simulink model "Assignment1"  (R2017b)
settings: Solver=FixedStepAuto  StartTime=0.0  StopTime=6  FixedStep=1e-3  RelTol=1e-3  EnableMultiTasking=on
undefined symbols (not defined in the file): D10, D11, D12, D2, D3, D4, D7, D8, D9, PTA0, PTA1, PTB23, PTB9, PTC3, PTC4, PTD0, PTD2, PTD3
libraries: frdmk64flib x12
settings Model: ExtModeTrigDuration=5  Creator=iannanla  LastModifiedBy=iannanla
settings DataIOCC: InspectSignalLogs=on
settings OptimizationCC: PassReuseOutputArgsAs=Individual arguments  MaxStackSize=64
settings DebuggingCC: ParameterTunabilityLossMsg=error
settings HardwareCC: ProdBitPerPointer=32  ProdBitPerSizeT=32  ProdBitPerPtrDiffT=32  ProdLargestAtomicInteger=Long  ProdLargestAtomicFloat=Double  ProdWordSize=32  ProdHWDeviceType=ARM Compatible->ARM Cortex
settings SFSimCC: MATLABDynamicMemAlloc=off
settings RTWCC: SystemTargetFile=ert.tlc  HardwareBoard=NXP FRDM-K64F  TemplateMakefile=ert_default_tmf  GenerateReport=on  Toolchain=GNU Tools for ARM Embedded Processors  IncludeHyperlinkInReport=on  LaunchReport=on  GenerateTraceInfo=on  GenerateTraceReport=on  GenerateTraceReportSl=on  GenerateTraceReportSf=on  GenerateTraceReportEml=on
settings CodeAppCC: ForceParamTrailComments=on  IgnoreCustomStorageClasses=off  OperatorAnnotations=on  SimulinkDataObjDesc=on  SFDataObjDesc=on  InsertBlockDesc=on

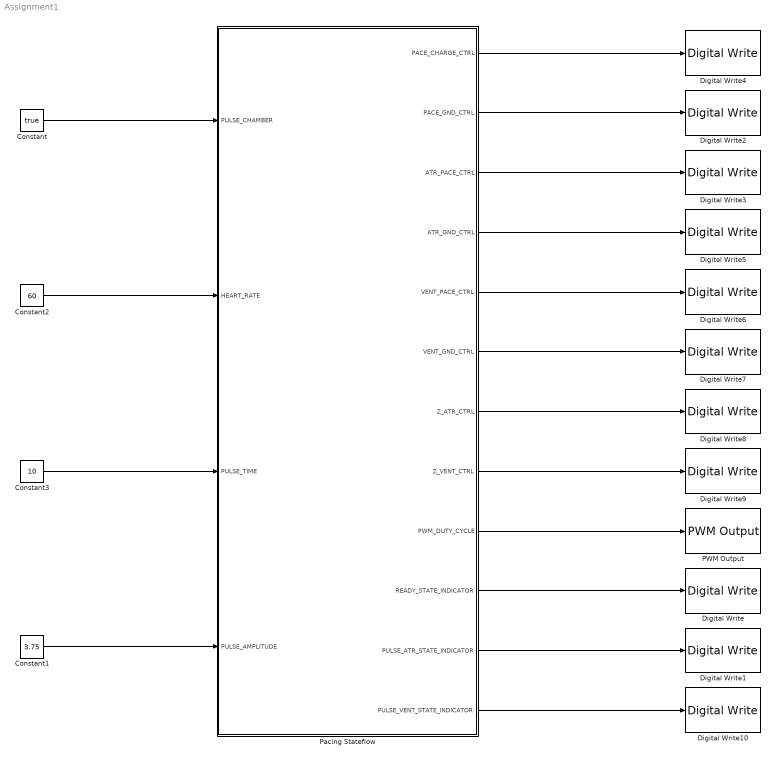
== system Assignment1 ==
  Constant : Constant  Value=true  OutDataTypeStr=boolean
  Constant1 : Constant  Value=3.75  OutDataTypeStr=int16
  Constant2 : Constant  Value=60  OutDataTypeStr=int16
  Constant3 : Constant  Value=10  OutDataTypeStr=int16
  Digital Write : frdmk64flib/Digital Write  Whichpin=RED_LED
      settings: SourceProductName=Simulink Coder Support Package for NXP FRDM-K64F Board
  Digital Write1 : frdmk64flib/Digital Write  Whichpin=BLUE_LED
      settings: SourceProductName=Simulink Coder Support Package for NXP FRDM-K64F Board
  Digital Write10 : frdmk64flib/Digital Write  Whichpin=GREEN_LED
      settings: SourceProductName=Simulink Coder Support Package for NXP FRDM-K64F Board
  Digital Write2 : frdmk64flib/Digital Write  Whichpin=PTD0 (D10)
      settings: SourceProductName=Simulink Coder Support Package for NXP FRDM-K64F Board
  Digital Write3 : frdmk64flib/Digital Write  Whichpin=PTA0 (D8)
      settings: SourceProductName=Simulink Coder Support Package for NXP FRDM-K64F Board
  Digital Write4 : frdmk64flib/Digital Write  Whichpin=PTB9 (D2)
      settings: SourceProductName=Simulink Coder Support Package for NXP FRDM-K64F Board
  Digital Write5 : frdmk64flib/Digital Write  Whichpin=PTD2 (D11)
      settings: SourceProductName=Simulink Coder Support Package for NXP FRDM-K64F Board
  Digital Write6 : frdmk64flib/Digital Write  Whichpin=PTC4 (D9)
      settings: SourceProductName=Simulink Coder Support Package for NXP FRDM-K64F Board
  Digital Write7 : frdmk64flib/Digital Write  Whichpin=PTD3 (D12)
      settings: SourceProductName=Simulink Coder Support Package for NXP FRDM-K64F Board
  Digital Write8 : frdmk64flib/Digital Write  Whichpin=PTB23 (D4)
      settings: SourceProductName=Simulink Coder Support Package for NXP FRDM-K64F Board
  Digital Write9 : frdmk64flib/Digital Write  Whichpin=PTC3 (D7)
      settings: SourceProductName=Simulink Coder Support Package for NXP FRDM-K64F Board
  PWM Output : frdmk64flib/PWM Output  Whichpin=PTA1 (D3)  InitialFrequency=1000  InitialDutyCycle=0
      settings: SourceProductName=Simulink Coder Support Package for NXP FRDM-K64F Board
  Pacing Stateflow : Stateflow chart  TreatAsAtomicUnit=on
  wires:
  Pacing Stateflow/1(PACE_CHARGE_CTRL) -> Digital Write4/1
  Pacing Stateflow/5(VENT_PACE_CTRL) -> Digital Write6/1
  Constant/1 -> Pacing Stateflow/1(PULSE_CHAMBER)
  Pacing Stateflow/2(PACE_GND_CTRL) -> Digital Write2/1
  Pacing Stateflow/3(ATR_PACE_CTRL) -> Digital Write3/1
  Pacing Stateflow/4(ATR_GND_CTRL) -> Digital Write5/1
  Pacing Stateflow/6(VENT_GND_CTRL) -> Digital Write7/1
  Pacing Stateflow/7(Z_ATR_CTRL) -> Digital Write8/1
  Pacing Stateflow/8(Z_VENT_CTRL) -> Digital Write9/1
  Constant2/1 -> Pacing Stateflow/2(HEART_RATE)
  Constant3/1 -> Pacing Stateflow/3(PULSE_TIME)
  Constant1/1 -> Pacing Stateflow/4(PULSE_AMPLITUDE)
  Pacing Stateflow/9(PWM_DUTY_CYCLE) -> PWM Output/1
  Pacing Stateflow/10(READY_STATE_INDICATOR) -> Digital Write/1
  Pacing Stateflow/11(PULSE_ATR_STATE_INDICATOR) -> Digital Write1/1
  Pacing Stateflow/12(PULSE_VENT_STATE_INDICATOR) -> Digital Write10/1

== stateflow chart Assignment1/Pacing Stateflow ==
  state READY_NEXT_PULSE
    entry:
    during:
    ATR_PACE_CTRL = false;
    VENT_PACE_CTRL = false;
    PWM_DUTY_CYCLE = 20*PULSE_AMPLITUDE;
    PACE_CHARGE_CTRL = true;
    PACE_GND_CTRL = true;
    Z_ATR_CTRL = false;
    Z_VENT_CTRL = false;
    ATR_GND_CTRL = true;
    VENT_GND_CTRL = true;
    READY_STATE_INDICATOR = true;
    exit:
    READY_STATE_INDICATOR = false;
  state PULSE_VENTRICLE
    entry:
    during:
    PACE_CHARGE_CTRL = false;
    PACE_GND_CTRL = false;
    ATR_PACE_CTRL = false;
    ATR_GND_CTRL = false;
    Z_ATR_CTRL = false;
    Z_VENT_CTRL = false;
    VENT_GND_CTRL = false;
    VENT_PACE_CTRL = true;
    PULSE_VENT_STATE_INDICATOR = true;
    exit:
    PULSE_VENT_STATE_INDICATOR = false;
  state PULSE_ATRIUM
    entry:
    during:
    PACE_CHARGE_CTRL = false;
    PACE_GND_CTRL = false;
    VENT_PACE_CTRL = false;
    VENT_GND_CTRL = false;
    Z_ATR_CTRL = false;
    Z_VENT_CTRL = false;
    ATR_GND_CTRL = false;
    ATR_PACE_CTRL = true;
    PULSE_ATR_STATE_INDICATOR = true;
    exit:
    PULSE_ATR_STATE_INDICATOR = false;
  READY_NEXT_PULSE -> PULSE_VENTRICLE [order 1] : [ (PULSE_CHAMBER==true) & after(((60000/HEART_RATE)-PULSE_TIME),msec)]
  READY_NEXT_PULSE -> PULSE_ATRIUM [order 2] : [(PULSE_CHAMBER==false) & after(500,msec)]
  (default) -> READY_NEXT_PULSE
  PULSE_VENTRICLE -> READY_NEXT_PULSE : [after(PULSE_TIME,msec)]
  PULSE_ATRIUM -> READY_NEXT_PULSE : [after (500,msec)]
  data: PACE_CHARGE_CTRL output boolean =false; PACE_GND_CTRL output boolean =false; ATR_PACE_CTRL output boolean =false; ATR_GND_CTRL output boolean =false; VENT_PACE_CTRL output boolean =false; VENT_GND_CTRL output boolean =false; Z_ATR_CTRL output boolean =false; Z_VENT_CTRL output boolean =false; PULSE_CHAMBER input boolean; HEART_RATE input int16; PULSE_TIME input int16; PULSE_AMPLITUDE input int16 [0..5]; PWM_DUTY_CYCLE output int16 [0..100]; READY_STATE_INDICATOR output boolean; PULSE_ATR_STATE_INDICATOR output boolean; PULSE_VENT_STATE_INDICATOR output boolean
